simulink model "PlanarInv"  (R2018a)
settings: Solver=VariableStepAuto  StartTime=0.0  StopTime=td  RelTol=1e-3
values from neighbouring files (symbols this model uses):
  KDinv = diag([kd1i kd2i])    [Parameter.m]    (also in modifyi.m)
  KPinv = diag([kp1i kp2i])    [Parameter.m]    (also in modifyi.m)
  qdi = input('')    [Parameter.m]    (also in modifyi.m = V)
  qiinv = input('')    [Parameter.m]
  tc = input('')    [Parameter.m]    (also in modifyi.m = V)
  Xd = input('')    [Parameter.m]    (also in modifyi.m = V)
  Xddotd = input('')    [Parameter.m]    (also in modifyi.m = V)
  Xdotd = input('')    [Parameter.m]    (also in modifyi.m = V)
undefined symbols (not defined in the file or in its folder): c11, c12, c21, DervJacobianA, Fkinematics, Fv, G1a, G1b, G2, InertiaMatrix, InverseJacobianA, JacobianA
settings Model: Creator=Amr  LastModifiedBy=Amr
settings SolverCC: MaxConsecutiveMinStep=5

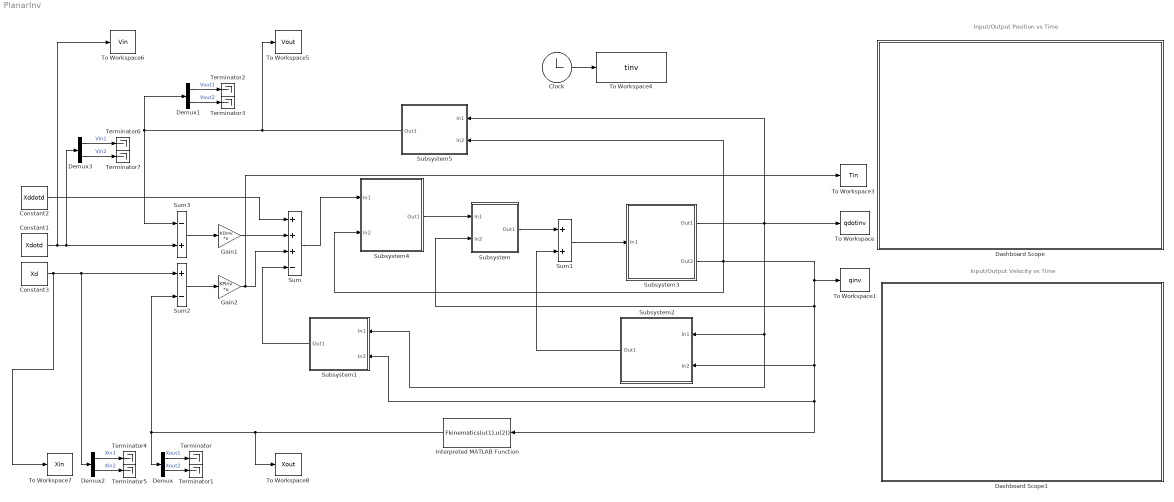
== system PlanarInv ==
  note: Input/Output Position vs Time
  note: Input/Output Velocity vs Time
  Clock : Clock
  Constant1 : Constant  Value=Xdotd  SampleTime=tc
  Constant2 : Constant  Value=Xddotd  SampleTime=tc
  Constant3 : Constant  Value=Xd  SampleTime=tc
  Dashboard Scope : Subsystem  DialogController=hmiCreateDDGDialog  IsWebBlock=on  mask(MWDashboardBlock){webBlockId=7bf5e091-c8a1-4e3f-a3de-79aaf862e1f5, webBlockType=sdiscope, ShowInitialText=on, HMISrcModelName=PlanarInv}
      mask prompts: webBlockId "WebBlock Id"; webBlockType "WebBlock Type"; HMISrcModelName "Source Model"
      mask help: SimulinkHMI:dialogs:HMIScopeDialogDesc
      mask Help: helpview([docroot '/mapfiles/simulink.map'], 'hmi_scope')
      mask Display:
      | if strcmp(get_param(bdroot(gcb),'BlockDiagramType'), 'library')
      |     image([(matlabroot) '/toolbox/simulink/hmi/icons/DashboardScope.png']);
      | end
  Dashboard Scope1 : Subsystem  DialogController=hmiCreateDDGDialog  IsWebBlock=on  mask(MWDashboardBlock){webBlockId=e652ddb0-efdc-4e3c-812f-868205cafe3c, webBlockType=sdiscope, ShowInitialText=on, HMISrcModelName=PlanarInv}
      mask prompts: webBlockId "WebBlock Id"; webBlockType "WebBlock Type"; HMISrcModelName "Source Model"
      mask help: SimulinkHMI:dialogs:HMIScopeDialogDesc
      mask Help: helpview([docroot '/mapfiles/simulink.map'], 'hmi_scope')
      mask Display:
      | if strcmp(get_param(bdroot(gcb),'BlockDiagramType'), 'library')
      |     image([(matlabroot) '/toolbox/simulink/hmi/icons/DashboardScope.png']);
      | end
  Demux{,1..3} (4 alike) : Demux  Outputs=2
  Gain1 : Gain  Gain=KDinv  Multiplication=Matrix(K*u)  SampleTime=tc
      mask Display: disp('KD')
  Gain2 : Gain  Gain=KPinv  Multiplication=Matrix(K*u)  SampleTime=tc
      mask Display: disp('KP')
  Interpreted MATLAB Function : MATLABFcn  MATLABFcn=Fkinematics(u(1),u(2))  OutputDimensions=2
      mask Display: disp('Forward Kinematics')
  Subsystem : Subsystem
      mask Display: disp('B(q)')
  Subsystem1 : Subsystem
      mask Display: disp('JA(q)dot')
  Subsystem2 : Subsystem
      mask Display: disp('n(q,qdot)')
  Subsystem3 : Subsystem
      mask Display: disp('Manipulator')
  Subsystem4 : Subsystem
      mask Display: disp('Inv(JA(q))')
  Subsystem5 : Subsystem
      mask Display: disp('JA(q)')
  Sum : Sum  Inputs=+++-
  Sum1 : Sum
  Sum2 : Sum  Inputs=+-
  Sum3 : Sum  Inputs=-+
  Terminator{,1..7} (8 alike) : Terminator
  To Workspace : ToWorkspace  VariableName=qdotinv  SampleTime=tc
      settings: MaxDataPoints=4001
  To Workspace1 : ToWorkspace  VariableName=qinv  SampleTime=tc
      settings: MaxDataPoints=4001
  To Workspace3 : ToWorkspace  VariableName=Tin  SampleTime=tc
      settings: MaxDataPoints=4001
  To Workspace4 : ToWorkspace  VariableName=tinv  SampleTime=tc
      settings: MaxDataPoints=4001
  To Workspace5 : ToWorkspace  VariableName=Vout  SampleTime=tc
      settings: MaxDataPoints=4001
  To Workspace6 : ToWorkspace  VariableName=Vin  SampleTime=tc
      settings: MaxDataPoints=4001
  To Workspace7 : ToWorkspace  VariableName=Xin  SampleTime=tc
      settings: MaxDataPoints=4001
  To Workspace8 : ToWorkspace  VariableName=Xout  SampleTime=tc
      settings: MaxDataPoints=4001
  wires:
  Sum1/1 -> Subsystem3/1(In1)
  Subsystem2/1(Out1) -> Sum1/2
  Subsystem/1(Out1) -> Sum1/1
  Demux3/2 -> Terminator7/1  "Vin2"
  Demux2/2 -> Terminator5/1  "Xin2"
  Demux/1 -> Terminator/1  "Xout1"
  Demux2/1 -> Terminator4/1  "Xin1"
  Constant2/1 -> Sum/1
  Demux1/1 -> Terminator2/1  "Vout1"
  Interpreted MATLAB Function/1 -> To Workspace8/1, Sum2/2, Demux/1
  Demux3/1 -> Terminator6/1  "Vin1"
  Gain1/1 -> Sum/2
  Constant1/1 -> To Workspace6/1, Demux3/1, Sum3/2
  Sum3/1 -> Gain1/1
  Sum2/1 -> Gain2/1
  Demux/2 -> Terminator1/1  "Xout2"
  Demux1/2 -> Terminator3/1  "Vout2"
  Gain2/1 -> To Workspace3/1, Sum/3
  Sum/1 -> Subsystem4/1(In1)
  Subsystem4/1(Out1) -> Subsystem/1(In1)
  Subsystem5/1(Out1) -> To Workspace5/1, Demux1/1, Sum3/1
  Constant3/1 -> To Workspace7/1, Sum2/1, Demux2/1
  Subsystem3/1(Out1) -> To Workspace/1, Subsystem5/1(In1), Subsystem1/1(In1), Subsystem2/1(In1)
  Subsystem3/2(Out2) -> To Workspace1/1, Subsystem1/2(In2), Interpreted MATLAB Function/1, Subsystem2/2(In2), Subsystem/2(In2), Subsystem5/2(In2), Subsystem4/2(In2)
  Subsystem1/1(Out1) -> Sum/4
  Clock/1 -> To Workspace4/1

== system PlanarInv/Dashboard Scope ==

== system PlanarInv/Dashboard Scope1 ==

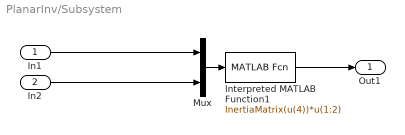
== system PlanarInv/Subsystem ==
  In1 : Inport
  In2 : Inport  Port=2
  Interpreted MATLAB Function1 : MATLABFcn  MATLABFcn=InertiaMatrix(u(4))*u(1:2)  OutputDimensions=2
  Mux : Mux  Inputs=2
  Out1 : Outport
  wires:
  Mux/1 -> Interpreted MATLAB Function1/1
  Interpreted MATLAB Function1/1 -> Out1/1
  In2/1 -> Mux/2
  In1/1 -> Mux/1

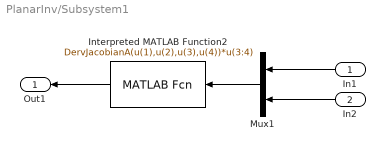
== system PlanarInv/Subsystem1 ==
  In1 : Inport
  In2 : Inport  Port=2
  Interpreted MATLAB Function2 : MATLABFcn  MATLABFcn=DervJacobianA(u(1),u(2),u(3),u(4))*u(3:4)  OutputDimensions=2
      mask Display: disp('JA(q)dot')
  Mux1 : Mux  Inputs=2
  Out1 : Outport
  wires:
  Mux1/1 -> Interpreted MATLAB Function2/1
  Interpreted MATLAB Function2/1 -> Out1/1
  In2/1 -> Mux1/2
  In1/1 -> Mux1/1

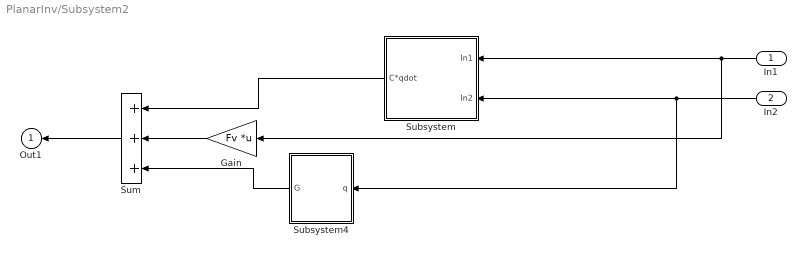
== system PlanarInv/Subsystem2 ==
  In1 : Inport
  In2 : Inport  Port=2
  Gain : Gain  Gain=Fv  Multiplication=Matrix(K*u)
      mask Display: disp('Friction')
  Subsystem : Subsystem
      mask Display: disp('C*qdot')
  Subsystem4 : Subsystem
      mask Display: disp('g(q)')
  Sum : Sum  Inputs=+++
  Out1 : Outport
  wires:
  In2/1 -> Subsystem/2(In2), Subsystem4/1(q)
  Subsystem4/1(G) -> Sum/3
  Sum/1 -> Out1/1
  Gain/1 -> Sum/2
  Subsystem/1(C*qdot) -> Sum/1
  In1/1 -> Gain/1, Subsystem/1(In1)

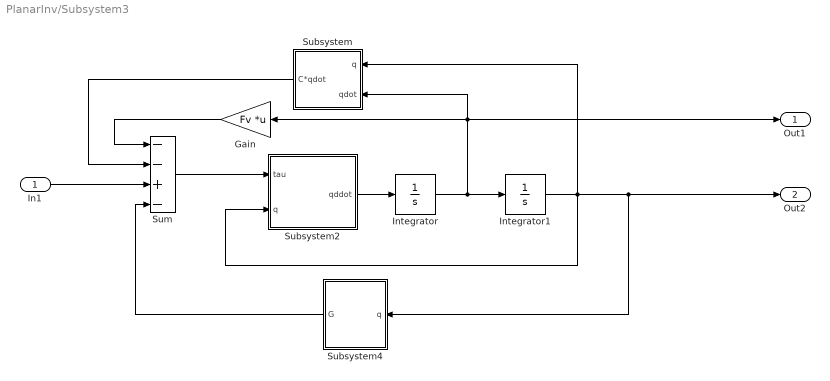
== system PlanarInv/Subsystem3 ==
  In1 : Inport
  Gain : Gain  Gain=Fv  Multiplication=Matrix(K*u)
      mask Display: disp('Friction')
  Integrator : Integrator  InitialCondition=qdi
  Integrator1 : Integrator  InitialCondition=qiinv
  Subsystem : Subsystem
      mask Display: disp('C*qdot')
  Subsystem2 : Subsystem
      mask Display: disp('inv(B(q))*tau')
  Subsystem4 : Subsystem
      mask Display: disp('g(q)')
  Sum : Sum  Inputs=--+-
  Out1 : Outport
  Out2 : Outport  Port=2
  wires:
  Subsystem/1(C*qdot) -> Sum/2
  Integrator1/1 -> Out2/1, Subsystem4/1(q), Subsystem2/2(q), Subsystem/1(q)
  Integrator/1 -> Out1/1, Gain/1, Subsystem/2(qdot), Integrator1/1
  Gain/1 -> Sum/1
  Sum/1 -> Subsystem2/1(tau)
  Subsystem2/1(qddot) -> Integrator/1
  Subsystem4/1(G) -> Sum/4
  In1/1 -> Sum/3

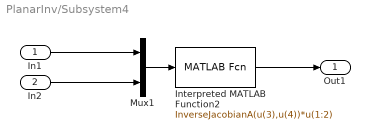
== system PlanarInv/Subsystem4 ==
  In1 : Inport
  In2 : Inport  Port=2
  Interpreted MATLAB Function2 : MATLABFcn  MATLABFcn=InverseJacobianA(u(3),u(4))*u(1:2)  OutputDimensions=2
      mask Display: disp('Inv(JA(q))')
  Mux1 : Mux  Inputs=2
  Out1 : Outport
  wires:
  Mux1/1 -> Interpreted MATLAB Function2/1
  In1/1 -> Mux1/1
  Interpreted MATLAB Function2/1 -> Out1/1
  In2/1 -> Mux1/2

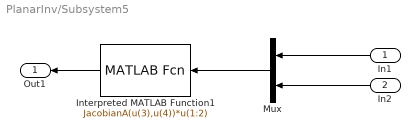
== system PlanarInv/Subsystem5 ==
  In1 : Inport
  In2 : Inport  Port=2
  Interpreted MATLAB Function1 : MATLABFcn  MATLABFcn=JacobianA(u(3),u(4))*u(1:2)  OutputDimensions=2
      mask Display: disp('JA(q)')
  Mux : Mux  Inputs=2
  Out1 : Outport
  wires:
  Mux/1 -> Interpreted MATLAB Function1/1
  In2/1 -> Mux/2
  Interpreted MATLAB Function1/1 -> Out1/1
  In1/1 -> Mux/1

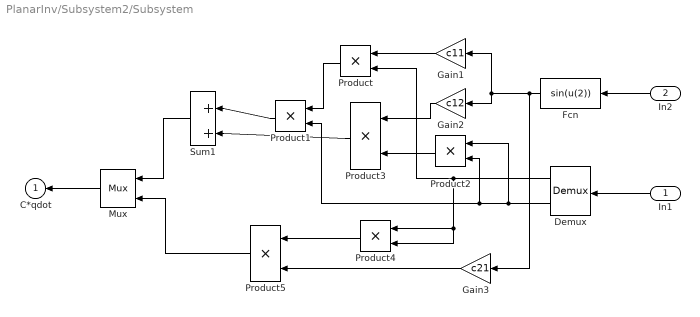
== system PlanarInv/Subsystem2/Subsystem ==
  In1 : Inport
  In2 : Inport  Port=2
  Demux : Demux  Outputs=2
      mask Display: disp('Demux')
  Fcn : Fcn  Expr=sin(u(2))
  Gain1 : Gain  Gain=c11
      mask Display: disp('c11')
  Gain2 : Gain  Gain=c12
      mask Display: disp('c12')
  Gain3 : Gain  Gain=c21
      mask Display: disp('c21')
  Mux : Mux  Inputs=2
      mask Display: disp('Mux')
  Product{,1..5} (6 alike) : Product
  Sum1 : Sum  Inputs=|++
  C*qdot : Outport
  wires:
  Product2/1 -> Product3/2
  Product/1 -> Product1/1
  Sum1/1 -> Mux/1
  Product4/1 -> Product5/1
  Fcn/1 -> Gain3/1, Gain2/1, Gain1/1
  Demux/2 -> Product2/2, Product1/2, Product2/1
  Mux/1 -> C*qdot/1
  Gain3/1 -> Product5/2
  Demux/1 -> Product/2, Product4/1, Product4/2
  Gain1/1 -> Product/1
  Product3/1 -> Sum1/2
  Gain2/1 -> Product3/1
  Product5/1 -> Mux/2
  Product1/1 -> Sum1/1
  In2/1 -> Fcn/1
  In1/1 -> Demux/1

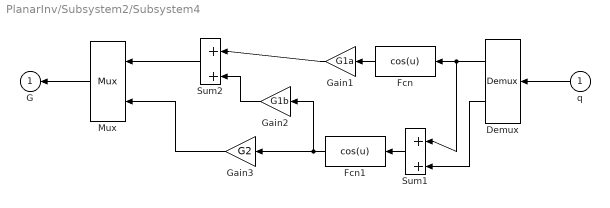
== system PlanarInv/Subsystem2/Subsystem4 ==
  q : Inport
  Demux : Demux  Outputs=2
      mask Display: disp('Demux')
  Fcn : Fcn  Expr=cos(u)
  Fcn1 : Fcn  Expr=cos(u)
  Gain1 : Gain  Gain=G1a
      mask Display: disp('G1a')
  Gain2 : Gain  Gain=G1b
      mask Display: disp('G1b')
  Gain3 : Gain  Gain=G2
      mask Display: disp('G2')
  Mux : Mux  Inputs=2
      mask Display: disp('Mux')
  Sum1 : Sum  Inputs=|++
  Sum2 : Sum  Inputs=|++
  G : Outport
  wires:
  Gain2/1 -> Sum2/2
  Fcn/1 -> Gain1/1
  Gain1/1 -> Sum2/1
  Demux/1 -> Fcn/1, Sum1/1
  Fcn1/1 -> Gain3/1, Gain2/1
  Gain3/1 -> Mux/2
  Demux/2 -> Sum1/2
  Sum1/1 -> Fcn1/1
  Sum2/1 -> Mux/1
  Mux/1 -> G/1
  q/1 -> Demux/1

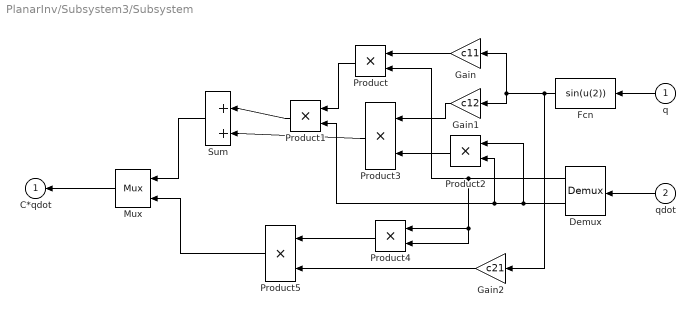
== system PlanarInv/Subsystem3/Subsystem ==
  q : Inport
  qdot : Inport  Port=2
  Demux : Demux  Outputs=2
      mask Display: disp('Demux')
  Fcn : Fcn  Expr=sin(u(2))
  Gain : Gain  Gain=c11
      mask Display: disp('c11')
  Gain1 : Gain  Gain=c12
      mask Display: disp('c12')
  Gain2 : Gain  Gain=c21
      mask Display: disp('c21')
  Mux : Mux  Inputs=2
      mask Display: disp('Mux')
  Product{,1..5} (6 alike) : Product
  Sum : Sum  Inputs=|++
  C*qdot : Outport
  wires:
  Demux/2 -> Product2/2, Product1/2, Product2/1
  Sum/1 -> Mux/1
  Product5/1 -> Mux/2
  Demux/1 -> Product/2, Product4/1, Product4/2
  Product4/1 -> Product5/1
  Fcn/1 -> Gain2/1, Gain1/1, Gain/1
  Gain2/1 -> Product5/2
  Product2/1 -> Product3/2
  Product1/1 -> Sum/1
  Product/1 -> Product1/1
  q/1 -> Fcn/1
  Gain1/1 -> Product3/1
  Product3/1 -> Sum/2
  qdot/1 -> Demux/1
  Mux/1 -> C*qdot/1
  Gain/1 -> Product/1

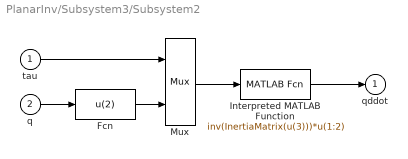
== system PlanarInv/Subsystem3/Subsystem2 ==
  tau : Inport
  q : Inport  Port=2
  Fcn : Fcn  Expr=u(2)
  Interpreted MATLAB Function : MATLABFcn  MATLABFcn=inv(InertiaMatrix(u(3)))*u(1:2)  OutputDimensions=2
  Mux : Mux  Inputs=[2,1]
      mask Display: disp('Mux')
  qddot : Outport
  wires:
  Mux/1 -> Interpreted MATLAB Function/1
  Interpreted MATLAB Function/1 -> qddot/1
  q/1 -> Fcn/1
  tau/1 -> Mux/1
  Fcn/1 -> Mux/2

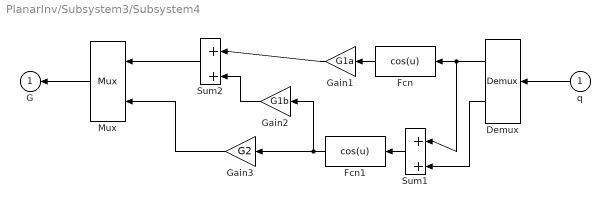
== system PlanarInv/Subsystem3/Subsystem4 ==
  q : Inport
  Demux : Demux  Outputs=2
      mask Display: disp('Demux')
  Fcn : Fcn  Expr=cos(u)
  Fcn1 : Fcn  Expr=cos(u)
  Gain1 : Gain  Gain=G1a
      mask Display: disp('G1a')
  Gain2 : Gain  Gain=G1b
      mask Display: disp('G1b')
  Gain3 : Gain  Gain=G2
      mask Display: disp('G2')
  Mux : Mux  Inputs=2
      mask Display: disp('Mux')
  Sum1 : Sum  Inputs=|++
  Sum2 : Sum  Inputs=|++
  G : Outport
  wires:
  Gain2/1 -> Sum2/2
  Fcn/1 -> Gain1/1
  Gain1/1 -> Sum2/1
  Demux/1 -> Fcn/1, Sum1/1
  Fcn1/1 -> Gain3/1, Gain2/1
  Gain3/1 -> Mux/2
  Demux/2 -> Sum1/2
  Sum1/1 -> Fcn1/1
  Sum2/1 -> Mux/1
  Mux/1 -> G/1
  q/1 -> Demux/1
